simulink model "V8_mdl_KF_imp"  (R2026a)
settings: Solver=ode45  StartTime=0  StopTime=1990  FixedStep=0.01  MaxStep=0.01
undefined symbols (not defined in the file): DiscIntNeverNeededParam, engineInertia, frontWheelMass, params, quarterCarMass, RAD2RPM, transmissionRatio, vehicle, vehicleMass, wheelRadius
libraries: matrix_library x2, V8SC_controls x2
settings Model: Creator=lholliday  LastModifiedBy=lholliday
settings SolverCC: InitialStep=0.01  ZeroCrossAlgorithm=Adaptive
settings DebuggingCC: IgnoredZcDiagnostic=none

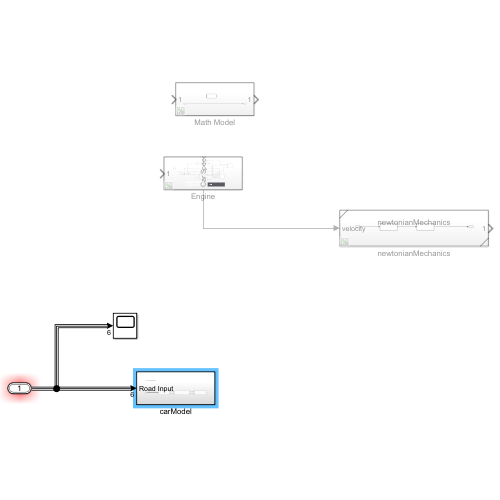
[thumbnail: Simulink's stored preview of the top-level diagram]
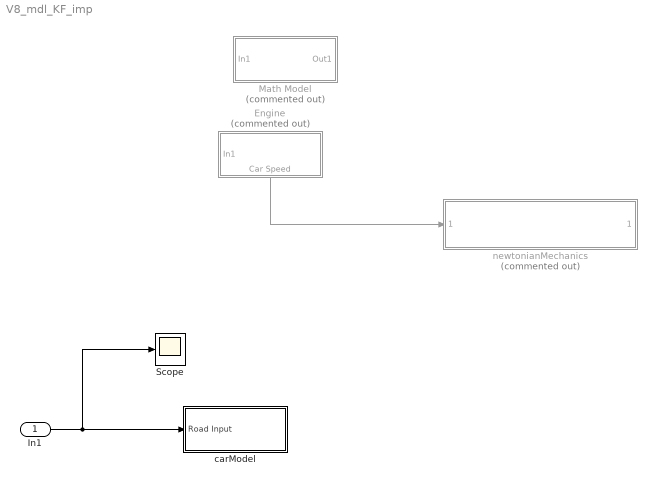
== system V8_mdl_KF_imp ==
  In1 : Inport  OutDataTypeStr=Bus: AugInputBus
  Engine : Subsystem  Commented=on
      settings: PortSchema="{\"entries\":[{\"content\":{\"sides\":[{\"content\":{\"connectorIds\":[\"In1\"]},\"type\":\"ConnectorPlacement.EquallySpacedRectSide\",\"uuid\":\"cadefebd-ad35-45dd-ae6a-9cccba43091e\"},{\"content\":{\"side\":\"RIGHT\"},\"type\":\"ConnectorPlacement.EquallySpacedRectSide\",\"uuid\":\"19d80bd4-267d-442e-b097-df40bf687d47\"},{\"content\":{\"side\":\"TOP\"},\"type\":\"ConnectorPlacement.EquallySpacedRectSide\",\"uuid\":\"6fb819b3-fb92-45d9-900f-1a7e7377e005\"},{\"content\":{\"connectorIds\":[\"Out1\"],\"side\":\"BOTTOM\"},\"type\":\"ConnectorPlacement.EquallySpacedRectSide\",\"uuid\":\"7f1958ad-d9a3-4585-8001-e48a895689d5\"}]},\"type\":\"ConnectorPlacement.EquallySpacedConnector\",\"uuid\":\"841cb558-8111-43be-8d99-0da8351c5108\"}],\"packageUris\":[\"http://schema.mathworks.com/mf0/Connector/R2020b\"],\"version\":\"1.0\"}"
  Math Model : Subsystem  Commented=on
  Scope : Scope
      settings: ActiveDisplayYMinimum=90.618291692113246  ActiveDisplayYMaximum=130.09592938047967  DataLoggingVariableName=ScopeData28
  carModel : Subsystem
  newtonianMechanics : Subsystem  Commented=on  ReferencedSubsystem=newtonianMechanics
  wires:
  Engine/1(Car Speed) -> newtonianMechanics/1
  In1/1 -> Scope/1, carModel/1(Road Input)

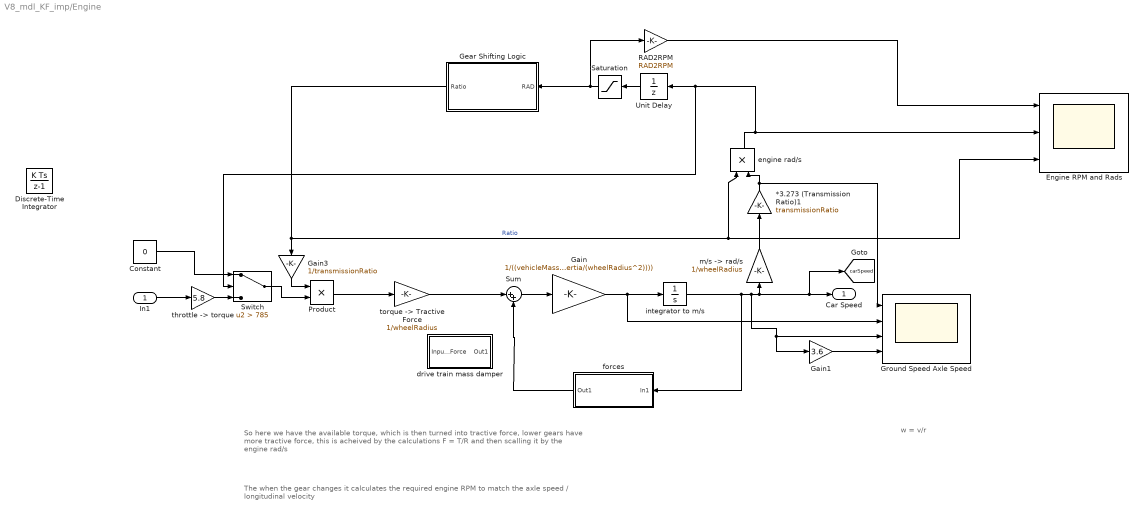
== system V8_mdl_KF_imp/Engine ==
  note: w = v/r
  note: The when the gear changes it calculates the required engine RPM to match the axle speed / longitudinal velocity
  note: So here we have the available torque, which is then turned into tractive force, lower gears have more tractive force, this is acheived by the calculations F = T/R and then scalling it by the engine rad/s
  In1 : Inport
  *3.273 (Transmission Ratio)1 : Gain  Gain=transmissionRatio
  Constant : Constant  Value=0
  Discrete-Time Integrator : DiscreteIntegrator  InitialConditionSource=external  SampleTime=-1  ICPrevOutput=DiscIntNeverNeededParam  ICPrevScaledInput=DiscIntNeverNeededParam
  Engine RPM and Rads : Scope  NumInputPorts=3
      settings: ActiveDisplayYMinimum=5459.4365717640658  ActiveDisplayYMaximum=8132.1776448532992
  Gain : Gain  Gain=1/((vehicleMass + (engineInertia/(wheelRadius^2))))
  Gain1 : Gain  Gain=3.6
  Gain3 : Gain  Gain=1/transmissionRatio
  Gear Shifting Logic : Subsystem
  Ground Speed Axle Speed : Scope  NumInputPorts=4
      settings: ActiveDisplayYMinimum=-98.141798139810533  ActiveDisplayYMaximum=883.27618325829508  DataLoggingVariableName=ScopeData5
  Product : Product
  RAD2RPM : Gain  Gain=RAD2RPM
  Saturation : Saturate  UpperLimit=7600  LowerLimit=0
  Sum : Sum  Inputs=|++
  Switch : Switch  Criteria=u2 > Threshold  Threshold=785  SaturateOnIntegerOverflow=off  InputSameDT=off
  Unit Delay : UnitDelay  SampleTime=-1
  drive train mass damper : Subsystem
  engine rad/s : Product
  forces : Subsystem
  integrator to m/s : Integrator
  "m/s -> rad/s" : Gain  Gain=1/wheelRadius
  "throttle -> torque" : Gain  Gain=5.8
  "torque -> Tractive Force" : Gain  Gain=1/wheelRadius
  Car Speed : Outport
  tag scope: carSpeed=global
  wires:
  In1/1 -> "throttle -> torque"/1
  Gain/1 -> Ground Speed Axle Speed/2, integrator to m/s/1
  forces/1(Out1) -> Sum/2
  Gear Shifting Logic/1(Ratio) -> Engine RPM and Rads/3, engine rad/s/1, Gain3/1  "Ratio"
  integrator to m/s/1 -> forces/1(In1), Gain1/1, Ground Speed Axle Speed/3, [carSpeed], Car Speed/1, "m/s -> rad/s"/1
  "m/s -> rad/s"/1 -> *3.273 (Transmission Ratio)1/1
  Unit Delay/1 -> Saturation/1
  Saturation/1 -> RAD2RPM/1, Gear Shifting Logic/1(RAD)
  Gain1/1 -> Ground Speed Axle Speed/4
  Product/1 -> "torque -> Tractive Force"/1
  engine rad/s/1 -> Switch/2, Unit Delay/1, Engine RPM and Rads/2
  RAD2RPM/1 -> Engine RPM and Rads/1
  *3.273 (Transmission Ratio)1/1 -> engine rad/s/2, Ground Speed Axle Speed/1
  Gain3/1 -> Product/1
  Sum/1 -> Gain/1
  Switch/1 -> Product/2
  "throttle -> torque"/1 -> Switch/3
  Constant/1 -> Switch/1
  "torque -> Tractive Force"/1 -> Sum/1

== system V8_mdl_KF_imp/Math Model ==
  In1 : Inport
  Stanley Controller : Subsystem
  Out1 : Outport
  wires:
  In1/1 -> Out1/1

== system V8_mdl_KF_imp/carModel ==
  note: X1 is the top portion
  Road Input : Inport
  Calculation : Subsystem
  Models : Subsystem
  State Estimation : Subsystem
  wires:
  Road Input/1 -> Models/1(Road In)
  Models/1(Model) -> State Estimation/1(Model)
  Models/2(Road Out) -> State Estimation/2(Road In)
  State Estimation/1(Estimation Station) -> Calculation/1(Estimation Station)
  State Estimation/2(Road Out) -> Calculation/2(Road In)

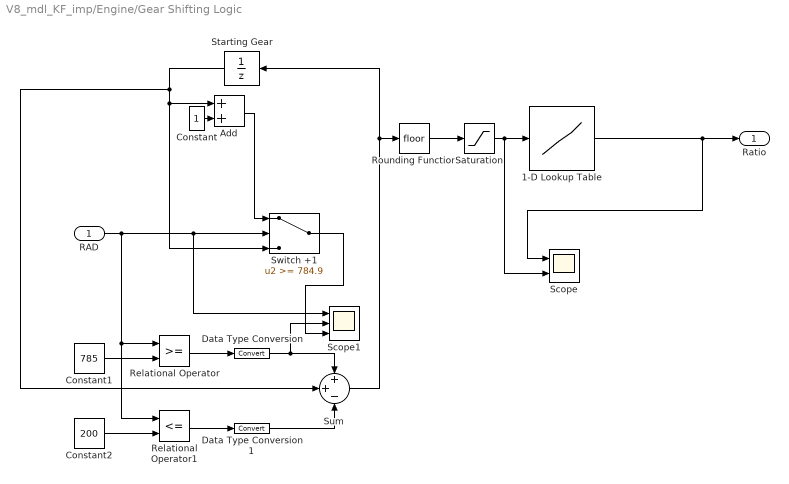
== system V8_mdl_KF_imp/Engine/Gear Shifting Logic ==
  RAD : Inport
  1-D Lookup Table : Lookup_n-D  NumberOfTableDimensions=1  BreakpointsForDimension1=[1;2;3;4;5;6]  Table=[2.5750000000000002;1.99;1.597;1.3300000000000001;1.143;1]  InternalRulePriority=Speed  RndMeth=Simplest
  Add : Sum
  Constant : Constant
  Constant1 : Constant  Value=785
  Constant2 : Constant  Value=200
  Data Type Conversion : DataTypeConversion  SaturateOnIntegerOverflow=off  RndMeth=Floor
  Data Type Conversion1 : DataTypeConversion  SaturateOnIntegerOverflow=off  RndMeth=Floor
  Relational Operator : RelationalOperator  OutDataTypeStr=fixdt(1,16)  RndMeth=Simplest  InputSameDT=off
  Relational Operator1 : RelationalOperator  Operator=<=  OutDataTypeStr=boolean  RndMeth=Simplest  InputSameDT=off
  Rounding Function : Rounding
  Saturation : Saturate  UpperLimit=6  LowerLimit=1
  Scope : Scope  NumInputPorts=2
      settings: ActiveDisplayYMinimum=0.80312500000000009  ActiveDisplayYMaximum=2.771875
  Scope1 : Scope  NumInputPorts=3
      settings: ActiveDisplayYMinimum=-98.326682289767959  ActiveDisplayYMaximum=884.94014060791187  DataLoggingVariableName=ScopeData3
  Starting Gear : UnitDelay  InitialCondition=1  SampleTime=-1
  Sum : Sum  Inputs=++-
  "Switch +1 " : Switch  Threshold=784.9  ZeroCross=off  SaturateOnIntegerOverflow=off  InputSameDT=off
  Ratio : Outport
  wires:
  Constant/1 -> Add/2
  Starting Gear/1 -> "Switch +1 "/3, Add/1, Sum/2
  "Switch +1 "/1 -> Scope1/3
  Saturation/1 -> Scope/2, 1-D Lookup Table/1
  Rounding Function/1 -> Saturation/1
  Add/1 -> "Switch +1 "/1
  1-D Lookup Table/1 -> Scope/1, Ratio/1
  Constant1/1 -> Relational Operator/2
  RAD/1 -> Relational Operator1/1, Relational Operator/1, "Switch +1 "/2, Scope1/1
  Constant2/1 -> Relational Operator1/2
  Relational Operator1/1 -> Data Type Conversion1/1
  Sum/1 -> Rounding Function/1, Starting Gear/1
  Relational Operator/1 -> Data Type Conversion/1
  Data Type Conversion/1 -> Scope1/2, Sum/1
  Data Type Conversion1/1 -> Sum/3

== system V8_mdl_KF_imp/Engine/drive train mass damper ==
  InputTractiveForce : Inport
  Add : Sum  Inputs=+--
  Damping Coeffienent : Gain  Gain=0.707
  DriveTrainMass : Gain  Gain=1/10
  Integrator : Integrator
  Integrator1 : Integrator
  Scope : Scope
      settings: ActiveDisplayYMinimum=-1  ActiveDisplayYMaximum=1  DataLoggingVariableName=ScopeData4
  Spring Stiffness : Gain  Gain=10
  Out1 : Outport
  wires:
  InputTractiveForce/1 -> Add/1
  Add/1 -> DriveTrainMass/1
  DriveTrainMass/1 -> Integrator/1
  Integrator/1 -> Damping Coeffienent/1, Integrator1/1
  Damping Coeffienent/1 -> Add/3
  Spring Stiffness/1 -> Add/2
  Integrator1/1 -> Spring Stiffness/1, Scope/1, Out1/1

== system V8_mdl_KF_imp/Engine/forces ==
  In1 : Inport
  Abs : Abs  SaturateOnIntegerOverflow=off
  Constant : Constant  Value=0
  Fcn1 : Fcn  Expr=u^2 * 1/2 * 1.225 * 0.05
  From : From
  Scope : Scope  NumInputPorts=2
      settings: ActiveDisplayYMinimum=-59.044453764161155  ActiveDisplayYMaximum=6.5604948626845712  DataLoggingVariableName=ScopeData2
  Sum : Sum  Inputs=|++
  rad to m/s1 : Gain  Gain=-1
  Out1 : Outport
  wires:
  In1/1 -> Fcn1/1, Scope/2
  Abs/1 -> rad to m/s1/1
  Fcn1/1 -> Sum/1
  Sum/1 -> Abs/1
  rad to m/s1/1 -> Scope/1, Out1/1
  Constant/1 -> Sum/2

== system V8_mdl_KF_imp/Math Model/Stanley Controller ==
  velocity : Inport
  crosstrack error : Inport  Port=2
  heading error : Inport  Port=3
  cross track gain : Inport  Port=4
  Add : Sum
  Product : Product
  Trigonometric Function : Trigonometry  Operator=atan2
  delta : Outport
  wires:
  crosstrack error/1 -> Product/1
  cross track gain/1 -> Product/2
  Product/1 -> Trigonometric Function/1
  heading error/1 -> Add/2
  velocity/1 -> Trigonometric Function/2
  Add/1 -> delta/1
  Trigonometric Function/1 -> Add/1

== system V8_mdl_KF_imp/carModel/Calculation ==
  Estimation Station : Inport
  Road In : Inport  Port=2
  Cx Calculation : Subsystem
  Out1 : Outport
  wires:
  Road In/1 -> Cx Calculation/1(In1)
  Cx Calculation/1(Out1) -> Out1/1

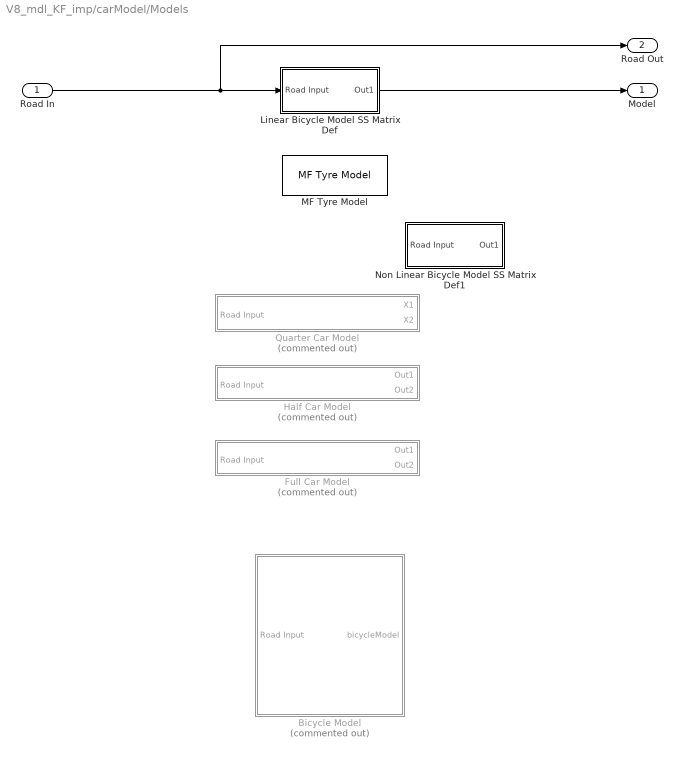
== system V8_mdl_KF_imp/carModel/Models ==
  Road In : Inport
  Bicycle Model : Subsystem  Commented=on
  Full Car Model : Subsystem  Commented=on
  Half Car Model : Subsystem  Commented=on
  Linear Bicycle Model SS Matrix Def : Subsystem
  MF Tyre Model : V8SC_controls/MF Tyre Model  SystemSampleTime=-1  VariantActivationTime=update diagram  EmptyChoice=off  PassThrough=off  PassThroughVariantControl=(default)  EmptyChoiceVariantControl=(default)  AllowFlexibleInterface=on  Latency=0  AutoFrameSizeCalculation=off
  Non Linear Bicycle Model SS Matrix Def1 : Subsystem
  Quarter Car Model : Subsystem  Commented=on
  Model : Outport
  Road Out : Outport  Port=2
  wires:
  Road In/1 -> Road Out/1, Linear Bicycle Model SS Matrix Def/1(Road Input)
  Linear Bicycle Model SS Matrix Def/1(Out1) -> Model/1

== system V8_mdl_KF_imp/carModel/State Estimation ==
  Model : Inport
  Road In : Inport  Port=2
  Estimator Creator : BusCreator  Inputs=1
  Linear Bicycle Model State Estimation : Subsystem
  Estimation Station : Outport
  Road Out : Outport  Port=2
  wires:
  Road In/1 -> Road Out/1, Linear Bicycle Model State Estimation/1(In1)
  Model/1 -> Linear Bicycle Model State Estimation/2(Model)
  Linear Bicycle Model State Estimation/2(Out2) -> Estimator Creator/1
  Estimator Creator/1 -> Estimation Station/1

== system V8_mdl_KF_imp/carModel/Calculation/Cx Calculation ==
  note: Requires a Differential equation to determin the resulting drag imposed on the system
  In1 : Inport
  Out1 : Outport
  wires:
  In1/1 -> Out1/1

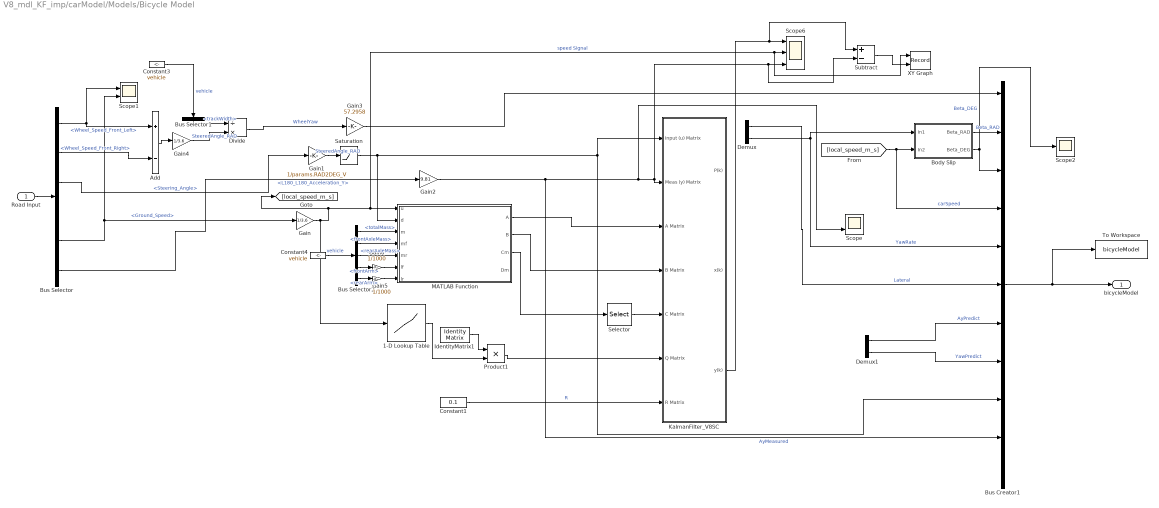
== system V8_mdl_KF_imp/carModel/Models/Bicycle Model ==
  Road Input : Inport
  1-D Lookup Table : Lookup_n-D  NumberOfTableDimensions=1  BreakpointsForDimension1=[0,23,23.1,70]  Table=[0.5,0.5,1,1]  InternalRulePriority=Speed  RndMeth=Simplest
  Add : Sum  Inputs=+-
  Body Slip : Subsystem
  Bus Creator1 : BusCreator  Inputs=11
  Bus Selector : BusSelector  OutputSignals=Wheel_Speed_Front_Left,Wheel_Speed_Front_Right,Steering_Angle,Acceleration_Y_Filt,Ground_Speed,L180_L180_Acceleration_Y
  Bus Selector1 : BusSelector  OutputSignals=ford.kinematics.body.trackWidth
  Bus Selector2 : BusSelector  OutputSignals=ford.bicycleModel.totalMass,ford.bicycleModel.frontAxleMass,ford.bicycleModel.rearAxleMass,ford.bicycleModel.frontArm,ford.bicycleModel.rearArm
  Constant1 : Constant  Value=0.1
  Constant3 : Constant  Value=vehicle  OutDataTypeStr=Bus: VehicleBus
  Constant4 : Constant  Value=vehicle  OutDataTypeStr=Bus: VehicleBus
  Demux : Demux  Outputs=2
  Demux1 : Demux  Outputs=2
  Divide : Product  Inputs=/*
  Gain : Gain  Gain=1/3.6
  Gain1 : Gain  Gain=1/params.RAD2DEG_V
  Gain2 : Gain  Gain=9.81
  Gain3 : Gain  Gain=57.2958
  Gain4 : Gain  Gain=1/3.6
  Gain5 : Gain  Gain=1/1000
  Gain6 : Gain  Gain=1/1000
  IdentityMatrix1 : IdentityMatrix  OutputDimensions=2
  KalmanFilter_V8SC : Subsystem  AncestorBlock=V8SC_controls/KalmanFilter_V8SC
  MATLAB Function : MATLAB Function  TreatAsAtomicUnit=on
  Product1 : Product
  Saturation : Saturate  UpperLimit=0.18  LowerLimit=-0.18
  Scope : Scope  NumInputPorts=2
      settings: ActiveDisplayYMinimum=-9.6462676122117177  ActiveDisplayYMaximum=14.273763279918205  DataLoggingVariableName=ScopeData10
  Scope1 : Scope  NumInputPorts=2
      settings: ActiveDisplayYMinimum=-12.241429873252471  ActiveDisplayYMaximum=242.92458668258504  DataLoggingVariableName=ScopeData9
  Scope2 : Scope
      settings: ActiveDisplayYMinimum=-0.87763523580666181  ActiveDisplayYMaximum=0.95550372211151358  DataLoggingVariableName=ScopeData12
  Scope6 : Scope  NumInputPorts=3
      settings: ActiveDisplayYMinimum=-0.60254405326556437  ActiveDisplayYMaximum=19.199492569813536  DataLoggingMaxPoints=200000  DataLoggingVariableName=ScopeData27
  Selector : Selector  NumberOfDimensions=2  InputPortWidth=3  IndexOptions=Index vector (dialog),Select all  Indices=1,1  OutputSizes=1,1
  Subtract : Sum  Inputs=+-
  To Workspace : ToWorkspace  VariableName=bicycleModel  SaveFormat=Timeseries  SampleTime=-1
  XY Graph : Record  NumPorts=2.0  FileSettingsInternal="{\"entries\":[{\"content\":{\"excelSettings\":{\"content\":{},\"type\":\"Streamout.ExcelSettings\"},\"parquetSettings\":{\"content\":{},\"type\":\"Streamout.ParquetSettings\"}},\"type\":\"Streamout.FileSettingStorage\",\"uuid\":\"\"}],\"packageUris\":[\"http:\\/\\/schema.mathworks.com\\/mf0\\/streamout_blocks\\/R2020a\"],\"version\":\"1.0\"}"  FrameSettings=[0, 0]  Layout=[1 1]  SignalsInternal="{\"entries\":[{\"content\":{\"signals\":[{\"content\":{\"blockPath\":[],\"dimensions\":[1],\"domain\":\"\",\"lineColor\":\"#a2142f\",\"plots\":[ 1 ],\"port\":1,\"signalID\":1,\"signalName\":\"speed Signal\"},\"type\":\"RecordBlkView.Signal\",\"uuid\":\"\"},{\"content\":{\"blockPath\":[],\"dimensions\":[1],\"domain\":\"\",\"lineColor\":\"#139fff\",\"plots\":[ 1 ],\"port\":2,\"signalID\":2,\"signalName\":\"Subtract\"},\"type\":\"RecordBlkView.Signal\",\"uuid\":\"\"}]},\"type\":\"RecordBlkView.InputSignals\",\"uuid\":\"\"}],\"packageUris\":[\"http:\\/\\/schema.mathworks.com\\/mf0\\/streamout_blocks\\/R2020a\"],\"version\":\"1.0\"}"  VisualizationBindings="{\"xyplotplugin\":{\"info\":[{\"series\":[{\"bindingParametersList\":[{\"parameter\":\"X-Axis\",\"signalID\":1,\"signalName\":\"speed Signal\"},{\"parameter\":\"Y-Axis\",\"signalID\":2,\"signalName\":\"Subtract\"}],\"seriesID\":0}],\"subplotID\":1}]}}"  CompatibilityTag=XY
  bicycleModel : Outport
  wires:
  Bus Selector/5 -> Gain/1, Scope1/2  "<Ground_Speed>"
  Bus Selector/3 -> Gain1/1  "<Steering_Angle>"
  Gain2/1 -> Scope/2, Subtract/2, Scope6/3, KalmanFilter_V8SC/2(Meas (y) Matrix), Bus Creator1/10  "AyMeasured"
  MATLAB Function/3(Cm) -> Selector/1
  Demux/1 -> Bus Creator1/6  "Lateral"
  Demux/2 -> Body Slip/1(In1), Bus Creator1/5  "YawRate"
  Bus Creator1/1 -> To Workspace/1, bicycleModel/1
  Body Slip/1(Beta_RAD) -> Bus Creator1/2  "Beta_RAD"
  [local_speed_m_s] -> Bus Creator1/4, Body Slip/2(In2)  "carSpeed"
  Body Slip/2(Beta_DEG) -> Scope2/1, Bus Creator1/3  "Beta_DEG"
  MATLAB Function/1(A) -> KalmanFilter_V8SC/3(A Matrix)
  MATLAB Function/2(B) -> KalmanFilter_V8SC/4(B Matrix)
  Gain1/1 -> Saturation/1  "SteeredAngle_RAD"
  Gain/1 -> XY Graph/1, Scope6/2, MATLAB Function/1(u), [local_speed_m_s], 1-D Lookup Table/1  "speed Signal"
  Bus Selector/6 -> Gain2/1  "<L180_L180_Acceleration_Y>"
  Divide/1 -> Gain3/1  "WheelYaw"
  Demux1/1 -> Bus Creator1/7  "AyPredict"
  Demux1/2 -> Bus Creator1/8  "YawPredict"
  ? -> Bus Creator1/11
  Road Input/1 -> Bus Selector/1
  Bus Selector/1 -> Add/1, Scope1/1  "<Wheel_Speed_Front_Left>"
  Bus Selector/2 -> Add/2  "<Wheel_Speed_Front_Right>"
  Constant3/1 -> Bus Selector1/1  "vehicle"
  Add/1 -> Gain4/1
  Bus Selector1/1 -> Divide/1  "<trackWidth>"
  Constant4/1 -> Bus Selector2/1  "vehicle"
  Bus Selector2/1 -> MATLAB Function/3(m)  "<totalMass>"
  Bus Selector2/2 -> MATLAB Function/4(mf)  "<frontAxleMass>"
  Bus Selector2/3 -> MATLAB Function/5(mr)  "<rearAxleMass>"
  Bus Selector2/4 -> Gain6/1  "<frontArm>"
  Bus Selector2/5 -> Gain5/1  "<rearArm>"
  Gain3/1 -> Bus Creator1/1
  Gain4/1 -> Divide/2  "SteeredAngle_RAD"
  Constant1/1 -> KalmanFilter_V8SC/7(R Matrix)  "R"
  IdentityMatrix1/1 -> Product1/1
  Product1/1 -> KalmanFilter_V8SC/6(Q Matrix)
  Selector/1 -> KalmanFilter_V8SC/5(C Matrix)
  Gain5/1 -> MATLAB Function/7(lr)
  Gain6/1 -> MATLAB Function/6(lf)
  Saturation/1 -> MATLAB Function/2(d), KalmanFilter_V8SC/1(Input (u) Matrix), Bus Creator1/9
  KalmanFilter_V8SC/3(y(k)) -> Subtract/1, Scope6/1
  1-D Lookup Table/1 -> Product1/2
  Subtract/1 -> XY Graph/2

== system V8_mdl_KF_imp/carModel/Models/Full Car Model ==
  Road Input : Inport
  Out1 : Outport
  Out2 : Outport  Port=2
  wires:
  Road Input/1 -> Out1/1

== system V8_mdl_KF_imp/carModel/Models/Half Car Model ==
  Road Input : Inport
  Out1 : Outport
  Out2 : Outport  Port=2
  wires:
  Road Input/1 -> Out1/1

== system V8_mdl_KF_imp/carModel/Models/Linear Bicycle Model SS Matrix Def ==
  Road Input : Inport
  BicycleModelBus : BusCreator  Inputs=3
  Bus Selector : BusSelector  OutputSignals=Ground_Speed,Steering_Angle
  Bus Selector2 : BusSelector  OutputSignals=ford.bicycleModel.totalMass,ford.bicycleModel.frontAxleMass,ford.bicycleModel.rearAxleMass,ford.bicycleModel.frontArm,ford.bicycleModel.rearArm
  Constant4 : Constant  Value=vehicle  OutDataTypeStr=Bus: VehicleBus
  Gain5 : Gain  Gain=1/1000
  Gain6 : Gain  Gain=1/1000
  MATLAB Function : MATLAB Function  TreatAsAtomicUnit=on
  Out1 : Outport
  wires:
  Gain6/1 -> MATLAB Function/6(lf)  "Front Arm"
  Bus Selector2/4 -> Gain6/1  "<frontArm>"
  Bus Selector2/1 -> MATLAB Function/3(m)  "<totalMass>"
  Bus Selector2/3 -> MATLAB Function/5(mr)  "<rearAxleMass>"
  Bus Selector2/5 -> Gain5/1  "<rearArm>"
  Constant4/1 -> Bus Selector2/1  "vehicle"
  Bus Selector2/2 -> MATLAB Function/4(mf)  "<frontAxleMass>"
  Bus Selector/1 -> MATLAB Function/1(u)  "<Ground_Speed>"
  MATLAB Function/1(A) -> BicycleModelBus/1  "A"
  MATLAB Function/4(Dm) -> ?
  Road Input/1 -> Bus Selector/1
  Bus Selector/2 -> MATLAB Function/2(d)  "<Steering_Angle>"
  MATLAB Function/3(Cm) -> BicycleModelBus/3  "C"
  Gain5/1 -> MATLAB Function/7(lr)  "Rear Arm"
  MATLAB Function/2(B) -> BicycleModelBus/2  "B"
  BicycleModelBus/1 -> Out1/1

== system V8_mdl_KF_imp/carModel/Models/Non Linear Bicycle Model SS Matrix Def1 ==
  Road Input : Inport
  BicycleModelBus : BusCreator  Inputs=3
  Bus Selector : BusSelector  OutputSignals=Ground_Speed,Steering_Angle
  Bus Selector2 : BusSelector  OutputSignals=ford.bicycleModel.totalMass,ford.bicycleModel.frontAxleMass,ford.bicycleModel.rearAxleMass,ford.bicycleModel.frontArm,ford.bicycleModel.rearArm
  Constant4 : Constant  Value=vehicle  OutDataTypeStr=Bus: VehicleBus
  Gain5 : Gain  Gain=1/1000
  Gain6 : Gain  Gain=1/1000
  MATLAB Function : MATLAB Function  TreatAsAtomicUnit=on
  Out1 : Outport
  wires:
  Gain6/1 -> MATLAB Function/6(lf)  "Front Arm"
  Bus Selector2/4 -> Gain6/1  "<frontArm>"
  Bus Selector2/1 -> MATLAB Function/3(m)  "<totalMass>"
  Bus Selector2/3 -> MATLAB Function/5(mr)  "<rearAxleMass>"
  Bus Selector2/5 -> Gain5/1  "<rearArm>"
  Constant4/1 -> Bus Selector2/1  "vehicle"
  Bus Selector2/2 -> MATLAB Function/4(mf)  "<frontAxleMass>"
  Bus Selector/1 -> MATLAB Function/1(u)  "<Ground_Speed>"
  MATLAB Function/1(A) -> BicycleModelBus/1  "A"
  MATLAB Function/4(Dm) -> ?
  Road Input/1 -> Bus Selector/1
  Bus Selector/2 -> MATLAB Function/2(d)  "<Steering_Angle>"
  MATLAB Function/3(Cm) -> BicycleModelBus/3  "C"
  Gain5/1 -> MATLAB Function/7(lr)  "Rear Arm"
  MATLAB Function/2(B) -> BicycleModelBus/2  "B"
  BicycleModelBus/1 -> Out1/1

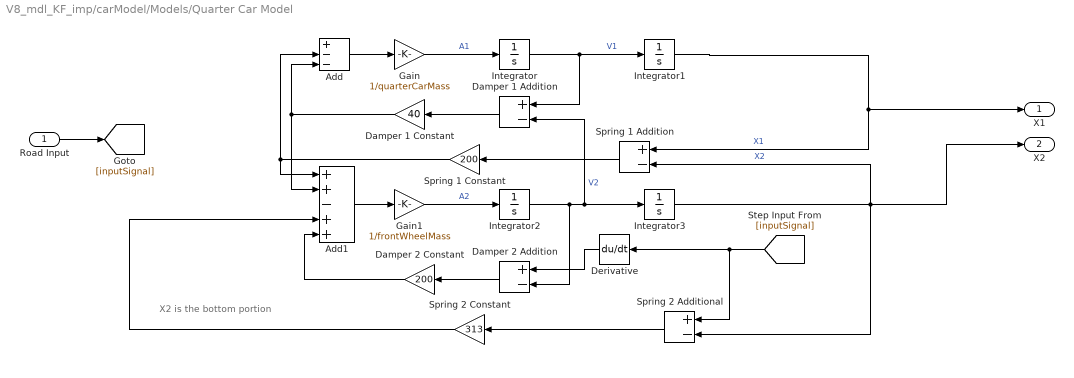
== system V8_mdl_KF_imp/carModel/Models/Quarter Car Model ==
  note: X2 is the bottom portion
  Road Input : Inport
  Add : Sum  Inputs=+--
  Add1 : Sum  Inputs=++-++
  Damper 1 Addition : Sum  Inputs=+-
  Damper 1 Constant : Gain  Gain=40
  Damper 2 Addition : Sum  Inputs=+-
  Damper 2 Constant : Gain  Gain=200
  Derivative : Derivative
  Gain : Gain  Gain=1/quarterCarMass
  Gain1 : Gain  Gain=1/frontWheelMass
  Integrator{,1..3} (4 alike) : Integrator
  Spring 1 Addition : Sum  Inputs=+-
  Spring 1 Constant : Gain  Gain=200
  Spring 2 Additional : Sum  Inputs=+-
  Spring 2 Constant : Gain  Gain=313
  X1 : Outport
  X2 : Outport  Port=2
  wires:
  Derivative/1 -> Damper 2 Addition/1
  Add/1 -> Gain/1
  Damper 2 Constant/1 -> Add1/5
  Add1/1 -> Gain1/1
  Damper 1 Constant/1 -> Add/3, Add1/2
  Spring 2 Additional/1 -> Spring 2 Constant/1
  [inputSignal] -> Spring 2 Additional/1, Derivative/1
  Integrator3/1 -> X2/1, Spring 2 Additional/2, Spring 1 Addition/2  "X2"
  Damper 2 Addition/1 -> Damper 2 Constant/1
  Spring 2 Constant/1 -> Add1/4
  Gain/1 -> Integrator/1  "A1"
  Integrator1/1 -> X1/1, Spring 1 Addition/1  "X1"
  Gain1/1 -> Integrator2/1  "A2"
  Integrator2/1 -> Damper 2 Addition/2, Damper 1 Addition/2, Integrator3/1  "V2"
  Integrator/1 -> Damper 1 Addition/1, Integrator1/1  "V1"
  Damper 1 Addition/1 -> Damper 1 Constant/1
  Spring 1 Constant/1 -> Add/2, Add1/1
  Spring 1 Addition/1 -> Spring 1 Constant/1
  Road Input/1 -> [inputSignal]

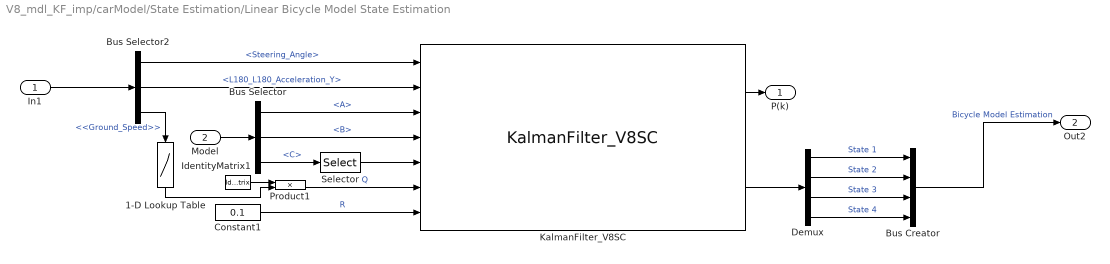
== system V8_mdl_KF_imp/carModel/State Estimation/Linear Bicycle Model State Estimation ==
  In1 : Inport
  Model : Inport  Port=2
  1-D Lookup Table : Lookup_n-D  NumberOfTableDimensions=1  BreakpointsForDimension1=[0,23,23.1,70]  Table=[0.5,0.5,1,1]  InternalRulePriority=Speed  RndMeth=Simplest
  Bus Creator : BusCreator  Inputs=4
  Bus Selector : BusSelector  OutputSignals=A,B,C
  Bus Selector2 : BusSelector  OutputSignals=Steering_Angle,L180_L180_Acceleration_Y,<Ground_Speed>
  Constant1 : Constant  Value=0.1
  Demux : Demux
  IdentityMatrix1 : IdentityMatrix  OutputDimensions=2
  KalmanFilter_V8SC : V8SC_controls/KalmanFilter_V8SC  SystemSampleTime=-1  VariantActivationTime=update diagram  EmptyChoice=off  PassThrough=off  PassThroughVariantControl=(default)  EmptyChoiceVariantControl=(default)  AllowFlexibleInterface=on  Latency=0  AutoFrameSizeCalculation=off
      settings: SourceProductName=V8SC controls
  Product1 : Product
  Selector : Selector  NumberOfDimensions=2  InputPortWidth=3  IndexOptions=Index vector (dialog),Select all  Indices=1,1  OutputSizes=1,1
  P(k) : Outport
  Out2 : Outport  Port=2
  wires:
  Model/1 -> Bus Selector/1
  Bus Selector2/3 -> 1-D Lookup Table/1  "<<Ground_Speed>>"
  Bus Selector/3 -> Selector/1  "<C>"
  Demux/4 -> Bus Creator/4  "State 4"
  Bus Selector/1 -> KalmanFilter_V8SC/3  "<A>"
  Bus Creator/1 -> Out2/1  "Bicycle Model Estimation"
  Constant1/1 -> KalmanFilter_V8SC/7  "R"
  Demux/1 -> Bus Creator/1  "State 1"
  KalmanFilter_V8SC/2 -> Demux/1
  Bus Selector/2 -> KalmanFilter_V8SC/4  "<B>"
  Product1/1 -> KalmanFilter_V8SC/6  "Q"
  Demux/2 -> Bus Creator/2  "State 2"
  1-D Lookup Table/1 -> Product1/2
  Bus Selector2/2 -> KalmanFilter_V8SC/2  "<L180_L180_Acceleration_Y>"
  Bus Selector2/1 -> KalmanFilter_V8SC/1  "<Steering_Angle>"
  Selector/1 -> KalmanFilter_V8SC/5
  Demux/3 -> Bus Creator/3  "State 3"
  IdentityMatrix1/1 -> Product1/1
  In1/1 -> Bus Selector2/1
  KalmanFilter_V8SC/1 -> P(k)/1

== system V8_mdl_KF_imp/carModel/Models/Bicycle Model/Body Slip ==
  In1 : Inport
  In2 : Inport  Port=2
  Constant : Constant  Value=params.RAD2DEG_V
  Product : Product
  Trigonometric Function : Trigonometry  Operator=atan2
  Beta_RAD : Outport
  Beta_DEG : Outport  Port=2
  wires:
  Trigonometric Function/1 -> Product/2, Beta_RAD/1  "Beta"
  In1/1 -> Trigonometric Function/1
  In2/1 -> Trigonometric Function/2
  Constant/1 -> Product/1
  Product/1 -> Beta_DEG/1  "Beta"

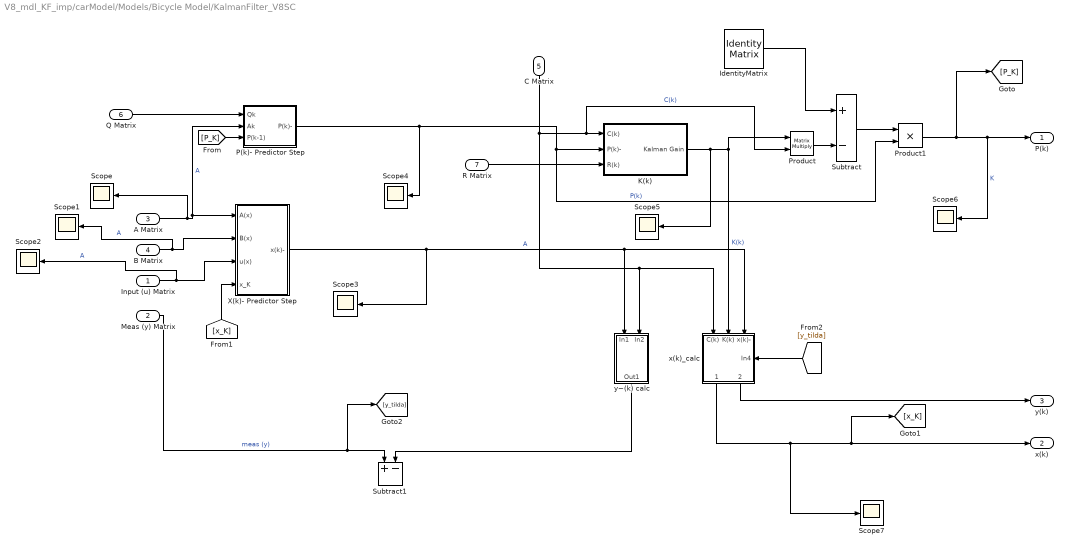
== system V8_mdl_KF_imp/carModel/Models/Bicycle Model/KalmanFilter_V8SC ==
  Input (u) Matrix : Inport
  Meas (y) Matrix : Inport  Port=2
  A Matrix : Inport  Port=3
  B Matrix : Inport  Port=4
  C Matrix : Inport  Port=5
  Q Matrix : Inport  Port=6
  R Matrix : Inport  Port=7
  IdentityMatrix : IdentityMatrix  OutputDimensions=2
  K(k) : Subsystem
  P(k)- Predictor Step : Subsystem
  Product : Product  Multiplication=Matrix(*)
  Product1 : Product
  Scope{,1..7} (8 alike) : Scope
      Scope settings: ActiveDisplayYMinimum=-0.91292616610272659  ActiveDisplayYMaximum=1.1447186134928031  DataLoggingVariableName=ScopeData16
      Scope1 settings: ActiveDisplayYMinimum=-76.902863771048189  ActiveDisplayYMaximum=81.800535438034714  DataLoggingVariableName=ScopeData17
      Scope2 settings: ActiveDisplayYMinimum=-0.039516708086627481  ActiveDisplayYMaximum=0.24986240109304589  DataLoggingVariableName=ScopeData18
      Scope3 settings: ActiveDisplayYMinimum=-8.5930774293256746  ActiveDisplayYMaximum=7.4203183990204549  DataLoggingVariableName=ScopeData19
      Scope4 settings: ActiveDisplayYMinimum=-5.2587260801662021E+306  ActiveDisplayYMaximum=1.0734804834239641E+307  DataLoggingVariableName=ScopeData16
      Scope5 settings: ActiveDisplayYMinimum=-0.82723024647713206  ActiveDisplayYMaximum=0.38370346141534284  DataLoggingVariableName=ScopeData17
      Scope6 settings: ActiveDisplayYMinimum=-1  ActiveDisplayYMaximum=1  DataLoggingVariableName=ScopeData18
      Scope7 settings: ActiveDisplayYMinimum=-1.2236133115950116  ActiveDisplayYMaximum=2.1293927293120229  DataLoggingVariableName=ScopeData16
  Subtract : Sum  Inputs=+-
  Subtract1 : Sum  Inputs=+-
  X(k)- Predictor Step : Subsystem
  x(k)_calc : Subsystem
      settings: PortSchema="{\"entries\":[{\"content\":{\"sides\":[{\"content\":{\"connectorIds\":[\"In1\",\"In2\",\"In3\"]},\"type\":\"ConnectorPlacement.EquallySpacedRectSide\",\"uuid\":\"9798f8d0-e1e5-4082-961b-6e38066891ac\"},{\"content\":{\"connectorIds\":[\"Out1\",\"Out2\"],\"side\":\"RIGHT\"},\"type\":\"ConnectorPlacement.EquallySpacedRectSide\",\"uuid\":\"85739a9d-0a70-4322-86b9-e4ddcc6280df\"},{\"content\":{\"side\":\"TOP\"},\"type\":\"ConnectorPlacement.EquallySpacedRectSide\",\"uuid\":\"b405db1d-aea8-46b4-b741-29e757833e0c\"},{\"content\":{\"connectorIds\":[\"In4\"],\"side\":\"BOTTOM\"},\"type\":\"ConnectorPlacement.EquallySpacedRectSide\",\"uuid\":\"98479f7e-2eaa-4af4-b745-0172a8769d4f\"}]},\"type\":\"ConnectorPlacement.EquallySpacedConnector\",\"uuid\":\"fea33aa2-baa4-4ea5-bbbc-a180d2a37d17\"}],\"packageUris\":[\"http://schema.mathworks.com/mf0/Connector/R2020b\"],\"version\":\"1.0\"}"
  y~(k) calc : Subsystem
  P(k) : Outport
  x(k) : Outport  Port=2
  y(k) : Outport  Port=3
  wires:
  [y_tilda] -> x(k)_calc/4(In4)
  R Matrix/1 -> K(k)/3(R(k))
  [x_K] -> X(k)- Predictor Step/4(x_K)
  [P_K] -> P(k)- Predictor Step/3(P(k-1))
  Meas (y) Matrix/1 -> Subtract1/1, [y_tilda]  "meas (y)"
  y~(k) calc/1(Out1) -> Subtract1/2
  x(k)_calc/1(x(k)_out) -> Scope7/1, x(k)/1, [x_K]
  Product1/1 -> Scope6/1, P(k)/1, [P_K]  "K"
  Subtract/1 -> Product1/1
  IdentityMatrix/1 -> Subtract/1
  Product/1 -> Subtract/2
  K(k)/1(Kalman Gain) -> Scope5/1, Product/1, x(k)_calc/2(K(k))  "K(k)"
  Q Matrix/1 -> P(k)- Predictor Step/1(Qk)
  P(k)- Predictor Step/1(P(k)-) -> Scope4/1, K(k)/2(P(k)-), Product1/2  "P(k)"
  C Matrix/1 -> Product/2, K(k)/1(C(k)), x(k)_calc/1(C(k)), y~(k) calc/2(In2)  "C(k)"
  A Matrix/1 -> Scope/1, P(k)- Predictor Step/2(Ak), X(k)- Predictor Step/1(A(x))  "A"
  B Matrix/1 -> Scope1/1, X(k)- Predictor Step/2(B(x))  "A"
  Input (u) Matrix/1 -> Scope2/1, X(k)- Predictor Step/3(u(x))  "A"
  X(k)- Predictor Step/1(x(k)-) -> Scope3/1, y~(k) calc/1(In1), x(k)_calc/3(x(k)-)  "A"
  x(k)_calc/2(y(k) out) -> y(k)/1

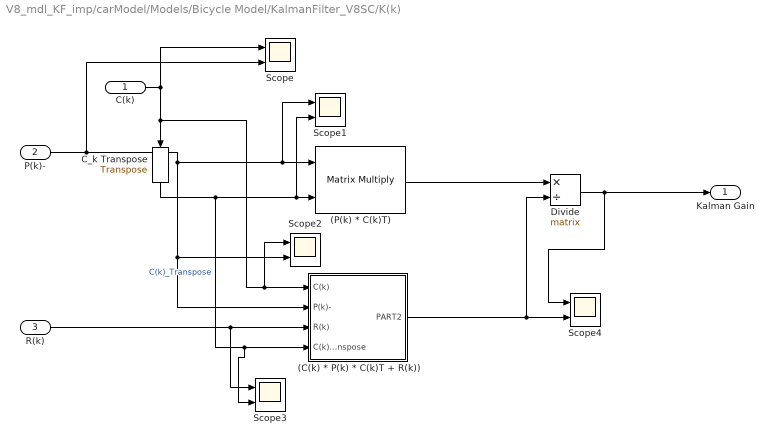
== system V8_mdl_KF_imp/carModel/Models/Bicycle Model/KalmanFilter_V8SC/K(k) ==
  C(k) : Inport
  P(k)- : Inport  Port=2
  R(k) : Inport  Port=3
  (C(k) * P(k) * C(k)T + R(k)) : Subsystem
  (P(k) * C(k)T) : Product  Multiplication=Matrix(*)
  C_k Transpose : matrix_library/Transpose
  Divide : Product  Inputs=*/  Multiplication=Matrix(*)
  Scope{,1..4} (5 alike) : Scope  NumInputPorts=2
      Scope settings: ActiveDisplayYMinimum=-1  ActiveDisplayYMaximum=1  DataLoggingVariableName=ScopeData16
      Scope1 settings: DataLoggingVariableName=ScopeData17
      Scope2 settings: DataLoggingVariableName=ScopeData18
      Scope3 settings: ActiveDisplayYMinimum=-1  ActiveDisplayYMaximum=1  DataLoggingVariableName=ScopeData19
      Scope4 settings: ActiveDisplayYMinimum=-13.081199890649827  ActiveDisplayYMaximum=2.4791057555640865  DataLoggingVariableName=ScopeData20
  Kalman Gain : Outport
  wires:
  Divide/1 -> Scope4/1, Kalman Gain/1
  (P(k) * C(k)T)/1 -> Divide/1
  R(k)/1 -> Scope3/1, (C(k) * P(k) * C(k)T + R(k))/3(R(k))
  (C(k) * P(k) * C(k)T + R(k))/1(PART2) -> Scope4/2, Divide/2
  C(k)/1 -> Scope2/1, (C(k) * P(k) * C(k)T + R(k))/1(C(k)), C_k Transpose/1, Scope/1
  C_k Transpose/1 -> Scope3/2, (C(k) * P(k) * C(k)T + R(k))/4(C(k)_Transpose), Scope1/2, (P(k) * C(k)T)/2  "C(k)_Transpose"
  P(k)-/1 -> (C(k) * P(k) * C(k)T + R(k))/2(P(k)-), Scope2/2, Scope1/1, (P(k) * C(k)T)/1, Scope/2

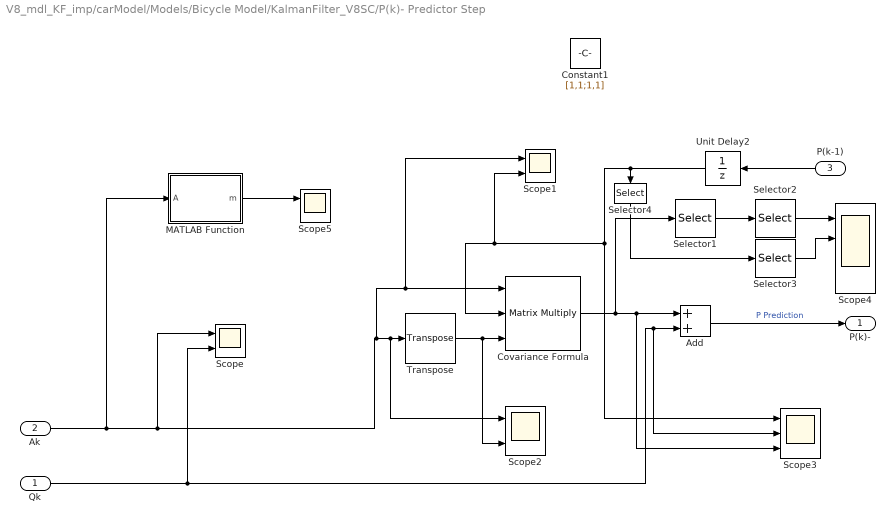
== system V8_mdl_KF_imp/carModel/Models/Bicycle Model/KalmanFilter_V8SC/P(k)- Predictor Step ==
  Qk : Inport
  Ak : Inport  Port=2
  P(k-1) : Inport  Port=3
  Add : Sum
  Constant1 : Constant  Value=[1,1;1,1]
  Covariance Formula : Product  Inputs=3  Multiplication=Matrix(*)
  MATLAB Function : MATLAB Function  TreatAsAtomicUnit=on
  Scope{,1..2,5} (4 alike) : Scope  NumInputPorts=2
      Scope settings: ActiveDisplayYMinimum=-124.93001065400131  ActiveDisplayYMaximum=41.410259316809892  DataLoggingVariableName=ScopeData16
      Scope1 settings: ActiveDisplayYMinimum=-0.911986572599679  ActiveDisplayYMaximum=1.1445335936858083  DataLoggingVariableName=ScopeData17
      Scope2 settings: ActiveDisplayYMinimum=-617.24111401067171  ActiveDisplayYMaximum=1202.37523413102  DataLoggingVariableName=ScopeData18
      Scope5 settings: ActiveDisplayYMinimum=0.63725957500490649  ActiveDisplayYMaximum=0.97326796602114662  DataLoggingVariableName=ScopeData26
  Scope3 : Scope  NumInputPorts=3
      settings: ActiveDisplayYMinimum=-5.8100421702498418E+305  ActiveDisplayYMaximum=8.9274255619736431E+304  DataLoggingVariableName=ScopeData19
  Scope4 : Scope  NumInputPorts=4
      settings: ActiveDisplayYMinimum=-2.3280355273851964E+303  ActiveDisplayYMaximum=1.5048330285378238E+303  DataLoggingVariableName=ScopeData25
  Selector1 : Selector  NumberOfDimensions=2  InputPortWidth=3  IndexOptions=Index vector (dialog),Select all  Indices=1,1  OutputSizes=1,1
  Selector2 : Selector  NumberOfDimensions=2  InputPortWidth=3  IndexOptions=Index vector (dialog),Index vector (dialog)  Indices=1,1  OutputSizes=1,1
  Selector3 : Selector  NumberOfDimensions=2  InputPortWidth=3  IndexOptions=Index vector (dialog),Index vector (dialog)  Indices=1,1  OutputSizes=1,1
  Selector4 : Selector  NumberOfDimensions=2  InputPortWidth=3  IndexOptions=Index vector (dialog),Select all  Indices=1,1  OutputSizes=1,1
  Transpose : matrix_library/Transpose
  Unit Delay2 : UnitDelay  InitialCondition=[1,1;1,1]  SampleTime=-1
  P(k)- : Outport
  wires:
  Covariance Formula/1 -> Selector1/1, Scope3/3, Add/1
  Qk/1 -> Scope/2, Scope3/2, Add/2
  Add/1 -> P(k)-/1  "P Prediction"
  Transpose/1 -> Scope2/2, Covariance Formula/3
  Unit Delay2/1 -> Selector4/1, Scope1/2, Covariance Formula/2, Scope3/1
  P(k-1)/1 -> Unit Delay2/1
  Selector1/1 -> Selector2/1
  Selector2/1 -> Scope4/1
  Selector3/1 -> Scope4/2
  Selector4/1 -> Selector3/1
  Ak/1 -> MATLAB Function/1(A), Scope/1, Scope2/1, Transpose/1, Scope1/1, Covariance Formula/1
  MATLAB Function/1(m) -> Scope5/1

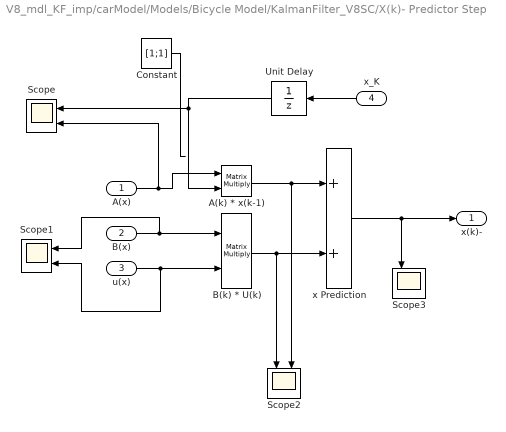
== system V8_mdl_KF_imp/carModel/Models/Bicycle Model/KalmanFilter_V8SC/X(k)- Predictor Step ==
  A(x) : Inport
  B(x) : Inport  Port=2
  u(x) : Inport  Port=3
  x_K : Inport  Port=4
  A(k) * x(k-1) : Product  Multiplication=Matrix(*)
  B(k) * U(k) : Product  Multiplication=Matrix(*)
  Constant : Constant  Value=[1;1]
  Scope{,1..3} (4 alike) : Scope  NumInputPorts=2
      Scope settings: ActiveDisplayYMinimum=-0.1896256836779612  ActiveDisplayYMaximum=0.23010664948459264  DataLoggingVariableName=ScopeData20
      Scope1 settings: ActiveDisplayYMinimum=-0.6278212197486237  ActiveDisplayYMaximum=0.7793239513320418  DataLoggingVariableName=ScopeData21
      Scope2 settings: ActiveDisplayYMinimum=-2.5171540368131966  ActiveDisplayYMaximum=22.654386331318772  DataLoggingVariableName=ScopeData22
      Scope3 settings: ActiveDisplayYMinimum=-1  ActiveDisplayYMaximum=1  DataLoggingVariableName=ScopeData23
  Unit Delay : UnitDelay  InitialCondition=[0;,0]  SampleTime=-1
  x Prediction : Sum
  x(k)- : Outport
  wires:
  x_K/1 -> Unit Delay/1
  A(x)/1 -> Scope/2, A(k) * x(k-1)/1
  Unit Delay/1 -> A(k) * x(k-1)/2, Scope/1
  x Prediction/1 -> Scope3/1, x(k)-/1
  B(x)/1 -> Scope1/1, B(k) * U(k)/1
  u(x)/1 -> Scope1/2, B(k) * U(k)/2
  A(k) * x(k-1)/1 -> Scope2/2, x Prediction/1
  B(k) * U(k)/1 -> Scope2/1, x Prediction/2
  Constant/1 -> ?

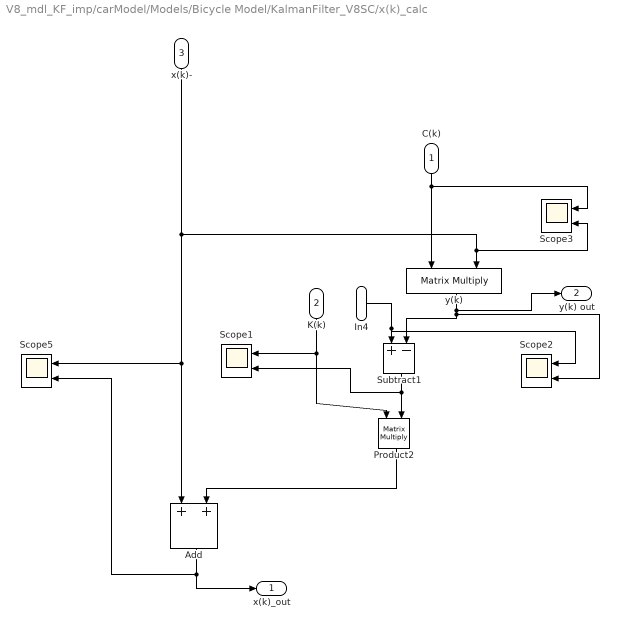
== system V8_mdl_KF_imp/carModel/Models/Bicycle Model/KalmanFilter_V8SC/x(k)_calc ==
  C(k) : Inport
  K(k) : Inport  Port=2
  x(k)- : Inport  Port=3
  In4 : Inport  Port=4
  Add : Sum
  Product2 : Product  Multiplication=Matrix(*)
  Scope{1..3,5} (4 alike) : Scope  NumInputPorts=2
      Scope1 settings: ActiveDisplayYMinimum=-2621.3263405902608  ActiveDisplayYMaximum=19024.847920273267  DataLoggingVariableName=ScopeData19
      Scope2 settings: ActiveDisplayYMinimum=-2621.3263405902608  ActiveDisplayYMaximum=19024.847920273267  DataLoggingVariableName=ScopeData17
      Scope3 settings: ActiveDisplayYMinimum=-2621.3263405902608  ActiveDisplayYMaximum=19024.847920273267  DataLoggingVariableName=ScopeData18
      Scope5 settings: ActiveDisplayYMinimum=-2621.3263405902608  ActiveDisplayYMaximum=19024.847920273267  DataLoggingVariableName=ScopeData19
  Subtract1 : Sum  Inputs=+-
  y(k) : Product  Multiplication=Matrix(*)
  x(k)_out : Outport
  y(k) out : Outport  Port=2
  wires:
  Add/1 -> Scope5/2, x(k)_out/1
  Subtract1/1 -> Scope1/2, Product2/2
  In4/1 -> Scope2/1, Subtract1/1
  C(k)/1 -> y(k)/1, Scope3/1
  Product2/1 -> Add/2
  x(k)-/1 -> Add/1, Scope5/1, y(k)/2, Scope3/2
  y(k)/1 -> y(k) out/1, Scope2/2, Subtract1/2
  K(k)/1 -> Scope1/1, Product2/1

== system V8_mdl_KF_imp/carModel/Models/Bicycle Model/KalmanFilter_V8SC/y~(k) calc ==
  In1 : Inport
  In2 : Inport  Port=2
  Product2 : Product  Multiplication=Matrix(*)
  Out1 : Outport
  wires:
  In2/1 -> Product2/1
  Product2/1 -> Out1/1
  In1/1 -> Product2/2

== system V8_mdl_KF_imp/carModel/Models/Bicycle Model/KalmanFilter_V8SC/K(k)/(C(k) * P(k) * C(k)T + R(k)) ==
  C(k) : Inport
  P(k)- : Inport  Port=2
  R(k) : Inport  Port=3
  C(k)_Transpose : Inport  Port=4
  Add1 : Sum
  Covariance Formula1 : Product  Inputs=3  Multiplication=Matrix(*)
  Scope : Scope  NumInputPorts=6
      settings: ActiveDisplayYMinimum=-31.493865136150596  ActiveDisplayYMaximum=1.379367419583799  DataLoggingVariableName=ScopeData24
  PART2 : Outport
  wires:
  Add1/1 -> Scope/5, PART2/1  "+"
  C(k)_Transpose/1 -> Covariance Formula1/3, Scope/3  "C(k)_Transpose"
  R(k)/1 -> Add1/2, Scope/4  "R(k)"
  C(k)/1 -> Covariance Formula1/1, Scope/1  "C(k)"
  Covariance Formula1/1 -> Scope/6, Add1/1  "Covariance"
  P(k)-/1 -> Covariance Formula1/2, Scope/2  "P(k)"

== matlab function V8_mdl_KF_imp/carModel/Models/Non Linear Bicycle Model SS Matrix Def1/MATLAB Function ==
  data: A output; B output; u input; d input; Cm output; Dm output; m input; mf input; mr input; lf input; lr input
function [A, B, Cm, Dm] = bicycleModelStateSpaceMatrix(u, d, m, mf, mr, lf, lr)

    u = max(u, 13);
    Iz  = mf*lf^2 + mr*lr^2;
    Caf = 150000;
    Car = 150000;

    A11 = -(2*Caf + 2*Car)/(m*u);
    A12 = -(u + (2*Caf*lf - 2*Car*lr)/(m*u));
    A21 =  (2*lf*Caf - 2*lr*Car)/(Iz*u);
    A22 = -(2*lf^2*Caf + 2*lr^2*Car)/(Iz*u);

    A_c = [A11, A12; A21, A22];         % continuous-time A
    B_c = [2*Caf/m; 2*Caf*lf/Iz] * d;   % continuous-time B

    % ---- Discretize before handing to the Kalman filter ----
    Ts = 0.01;    % <-- set this to your model's actual sample time
    A  = eye(2) + A_c*Ts;    % simple Euler discretization
    B  = B_c*Ts;

    % Kalman measurement matrix for ay — built from the CONTINUOUS A11/A12,
    % since Ay is a physical (continuous) measurement equation, not a state
    Cm = [A11, (A12+u); 0, 1];
    Dm = [2*Caf/m; 0];
end

== matlab function V8_mdl_KF_imp/carModel/Models/Linear Bicycle Model SS Matrix Def/MATLAB Function ==
  data: A output; B output; u input; d input; Cm output; Dm output; m input; mf input; mr input; lf input; lr input
function [A, B, Cm, Dm] = bicycleModelStateSpaceMatrix(u, d, m, mf, mr, lf, lr)

    u = max(u, 13);
    Iz  = mf*lf^2 + mr*lr^2;
    Caf = 150000;
    Car = 150000;

    A11 = -(2*Caf + 2*Car)/(m*u);
    A12 = -(u + (2*Caf*lf - 2*Car*lr)/(m*u));
    A21 =  (2*lf*Caf - 2*lr*Car)/(Iz*u);
    A22 = -(2*lf^2*Caf + 2*lr^2*Car)/(Iz*u);

    A_c = [A11, A12; A21, A22];         % continuous-time A
    B_c = [2*Caf/m; 2*Caf*lf/Iz] * d;   % continuous-time B

    % ---- Discretize before handing to the Kalman filter ----
    Ts = 0.01;    % <-- set this to your model's actual sample time
    A  = eye(2) + A_c*Ts;    % simple Euler discretization
    B  = B_c*Ts;

    % Kalman measurement matrix for ay — built from the CONTINUOUS A11/A12,
    % since Ay is a physical (continuous) measurement equation, not a state
    Cm = [A11, (A12+u); 0, 1];
    Dm = [2*Caf/m; 0];
end

== matlab function V8_mdl_KF_imp/carModel/Models/Bicycle Model/KalmanFilter_V8SC/P(k)- Predictor Step/MATLAB Function ==
  data: A input; m output
function m = maxEig(A)
    m = max(abs(eig(A)));
end

== matlab function V8_mdl_KF_imp/carModel/Models/Bicycle Model/MATLAB Function ==
  data: A output; B output; u input; d input; Cm output; Dm output; m input; mf input; mr input; lf input; lr input
function [A, B, Cm, Dm] = bicycleModelStateSpaceMatrix(u, d, m, mf, mr, lf, lr)

    u = max(u, 13);
    Iz  = mf*lf^2 + mr*lr^2;
    Caf = 150000;
    Car = 150000;

    A11 = -(2*Caf + 2*Car)/(m*u);
    A12 = -(u + (2*Caf*lf - 2*Car*lr)/(m*u));
    A21 =  (2*lf*Caf - 2*lr*Car)/(Iz*u);
    A22 = -(2*lf^2*Caf + 2*lr^2*Car)/(Iz*u);

    A_c = [A11, A12; A21, A22];         % continuous-time A
    B_c = [2*Caf/m; 2*Caf*lf/Iz] * d;   % continuous-time B

    % ---- Discretize before handing to the Kalman filter ----
    Ts = 0.01;    % <-- set this to your model's actual sample time
    A  = eye(2) + A_c*Ts;    % simple Euler discretization
    B  = B_c*Ts;

    % Kalman measurement matrix for ay — built from the CONTINUOUS A11/A12,
    % since Ay is a physical (continuous) measurement equation, not a state
    Cm = [A11, (A12+u); 0, 1];
    Dm = [2*Caf/m; 0];
end
